simulink model "super_etat"  (R2020a)
settings: Solver=VariableStepAuto  StartTime=0.0  StopTime=10.0  RelTol=1e-3
settings Model: Creator=ivanl  LastModifiedBy=ivanl

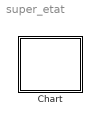
== system super_etat ==
  Chart : Stateflow chart  TreatAsAtomicUnit=on

== stateflow chart super_etat/Chart ==
  state Super_etat_2
    state sous_etat_2_1
    state sous_etat_2_2
    (default) -> sous_etat_2_1
    sous_etat_2_1 -> sous_etat_2_2 : [l==3]
    sous_etat_2_2 -> sous_etat_2_1 : [after(5,s)]
  state Super_etat_1
    state sous_etat_1_1
    state sous_etat_1_2
    (default) -> sous_etat_1_1
    sous_etat_1_1 -> sous_etat_1_2 [order 1] : [a<25]
    sous_etat_1_2 -> sous_etat_1_1 : [a>25]
  (default) -> Super_etat_1
  sous_etat_1_1 -> sous_etat_2_2 [order 2] : [default==1]
